simulink model "tuned"  (R2021a)
settings: Solver=VariableStepAuto  StartTime=0.0  StopTime=20  RelTol=1e-3
values from neighbouring files (symbols this model uses):
  A = processo.A    [esercizio1.m]
  B = processo.B    [esercizio1.m]
  C = processo.C    [esercizio1.m]
  D = processo.D    [esercizio1.m]
  I_PI_analogico_tuned = 0.325410877804267    (= 0.325410877804)    [esercizio1.m]
  I_PI_digitale_tuned = 0.28478840442912    (= 0.284788404429)    [esercizio1.m]
  I_PID_analogico_tuned = 0.279951410984123    (= 0.279951410984)    [esercizio1.m]
  I_PID_digitale_tuned = 0.172208500364823    (= 0.172208500365)    [esercizio1.m]
  KP_P = 0.5*Kcr    (= 2.15517241379)    [esercizio1.m]
  KP_P_analogico_tuned = 1.47219531686421    (= 1.47219531686)    [esercizio1.m]
  KP_P_digitale_tuned = 1.47219531686421    (= 1.47219531686)    [esercizio1.m]
  KP_PI = 0.45*Kcr    (= 1.93965517241)    [esercizio1.m]
  KP_PI_analogico_tuned = 1.47593963796892    (= 1.47593963797)    [esercizio1.m]
  KP_PI_digitale_tuned = 1.4003674925568    (= 1.40036749256)    [esercizio1.m]
  KP_PID = 0.6*Kcr    (= 2.58620689655)    [esercizio1.m]
  KP_PID_analogico_tuned = 1.9364815341473    (= 1.93648153415)    [esercizio1.m]
  KP_PID_digitale_tuned = 1.83497063890365    (= 1.8349706389)    [esercizio1.m]
  N = 100    [esercizio1.m]
  T = ta/40    [esercizio1.m]
  ta = 3*cost_temp_polo_dominante    [esercizio1.m]
  TD_PID = 0.12*Tcr    (= 0.24)    [esercizio1.m]
  TD_PID_analogico_tuned = 0.0554825984150835    (= 0.0554825984151)    [esercizio1.m]
  TD_PID_digitale_tuned = 0.0992484035615046    (= 0.0992484035615)    [esercizio1.m]
  TI_PI = 0.85*Tcr    (= 1.7)    [esercizio1.m]
  TI_PID = 0.5*Tcr    (= 1)    [esercizio1.m]
libraries: pid_lib x6
settings Model: Creator=Giorgio  LastModifiedBy=Giorgio

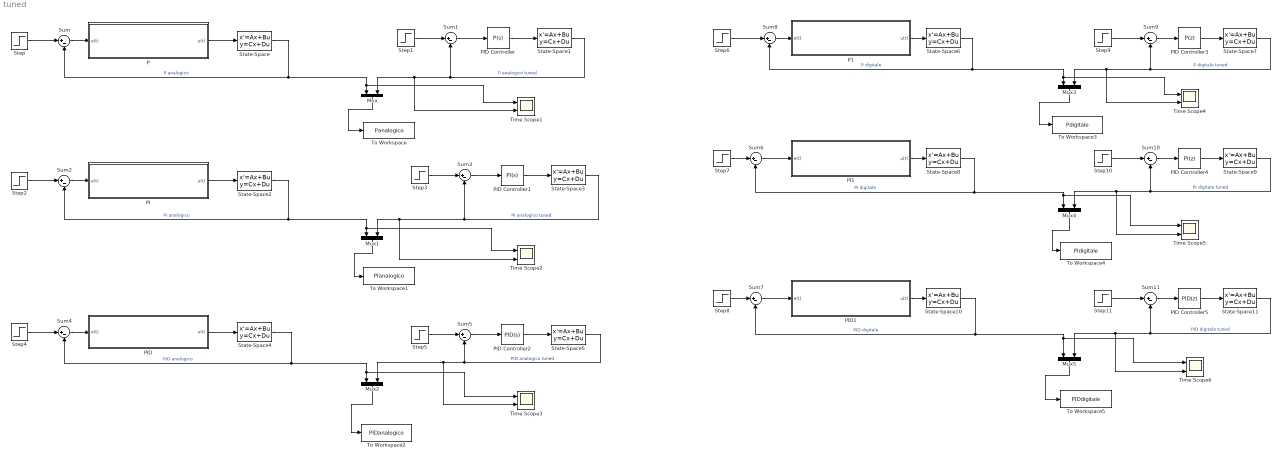
== system tuned ==
  Mux{,1..5} (6 alike) : Mux  Inputs=2
  P : Subsystem
  P1 : Subsystem
  PI : Subsystem
  PI1 : Subsystem
  PID : Subsystem
  PID Controller : pid_lib/PID Controller  Controller=P  Form=Ideal  TimeDomain=Continuous-time  UseExternalTs=off  SampleTime=-1  IntegratorMethod=Forward Euler  FilterMethod=Forward Euler  ControllerParametersSource=internal  P=KP_P_analogico_tuned  I=1  D=0  UseFilter=on  N=100  TunerSelectOption=Transfer Function Based (PID Tuner App)  InitialConditionSource=internal  InitialConditionForIntegrator=0  InitialConditionForFilter=0  DifferentiatorICPrevScaledInput=0  ExternalReset=none  TrackingMode=off  Kt=1  LimitOutput=off  SatLimitsSource=internal  UpperSaturationLimit=inf  LowerSaturationLimit=-inf  LinearizeAsGain=on  AntiWindupMode=none  Kb=1  POutMin=[]  POutMax=[]  IOutMin=[]  IOutMax=[]  DOutMin=[]  DOutMax=[]  NOutMin=[]  NOutMax=[]  SumOutMin=[]  SumOutMax=[]  SaturationOutMin=[]  SaturationOutMax=[]  PParamMin=[]  PParamMax=[]  IParamMin=[]  IParamMax=[]  DParamMin=[]  DParamMax=[]  NParamMin=[]  NParamMax=[]  KbParamMin=[]  KbParamMax=[]  KtParamMin=[]  KtParamMax=[]  KbOutMin=[]  KbOutMax=[]  KtOutMin=[]  KtOutMax=[]  IntegratorOutMin=[]  IntegratorOutMax=[]  FilterOutMin=[]  FilterOutMax=[]  SumI1OutMin=[]  SumI1OutMax=[]  SumI2OutMin=[]  SumI2OutMax=[]  SumI3OutMin=[]  SumI3OutMax=[]  SumI4OutMin=[]  SumI4OutMax=[]  SumDOutMin=[]  SumDOutMax=[]  DifferentiatorOutMin=[]  DifferentiatorOutMax=[]  FilterDiffOutCoefMin=[]  FilterDiffOutCoefMax=[]  ReciprocalOutMin=[]  ReciprocalOutMax=[]  SumDenOutMin=[]  SumDenOutMax=[]  SumNumOutMin=[]  SumNumOutMax=[]  DivideOutMin=[]  DivideOutMax=[]  UdiffTsProdOutMin=[]  UdiffTsProdOutMax=[]  NTsProdOutMin=[]  NTsProdOutMax=[]  UintegralTsProdOutMin=[]  UintegralTsProdOutMax=[]  UngainTsProdOutMin=[]  UngainTsProdOutMax=[]  IntegratorContinuousStateAttributes=''  IntegratorStateMustResolveToSignalObject=off  IntegratorRTWStateStorageClass=Auto  FilterContinuousStateAttributes=''  FilterStateMustResolveToSignalObject=off  FilterRTWStateStorageClass=Auto  ParallelPVariant=InternalParameters  IdealPVariant=Disabled  IVariant=Disabled  DVariant=Disabled  IntegratorVariant=Disabled  SatVariant=Disabled  AWVariant=Disabled  PCopyVariant=Disabled  TRVariant=Disabled  FdbkBlocksVariant=Forward  IdealPFdbkVariant=Disabled  SatFdbkVariant=Disabled  DerivativeFilterVariant=Disabled  NVariant=Disabled  NCopyVariant=Disabled_SignalSpec  FilterICVariant=Disabled  IntegratorICVariant=Disabled  ExternalResetVariant=Disabled  TRSumVariant=Passthrough  SumFdbkVariant=Disabled  SumVariant=Passthrough_P  TsampFilterVariant=InternalTs  TsampNgainVariant=Passthrough  TsampIntegralVariant=Disabled_SignalSpec  ExternalSaturationOutDataTypeStr=Inherit: Same as second input
  PID Controller1 : pid_lib/PID Controller  Controller=PI  Form=Ideal  TimeDomain=Continuous-time  UseExternalTs=off  SampleTime=-1  IntegratorMethod=Forward Euler  FilterMethod=Forward Euler  ControllerParametersSource=internal  P=KP_PI_analogico_tuned  I=I_PI_analogico_tuned  D=0  UseFilter=on  N=100  TunerSelectOption=Transfer Function Based (PID Tuner App)  InitialConditionSource=internal  InitialConditionForIntegrator=0  InitialConditionForFilter=0  DifferentiatorICPrevScaledInput=0  ExternalReset=none  TrackingMode=off  Kt=1  LimitOutput=off  SatLimitsSource=internal  UpperSaturationLimit=inf  LowerSaturationLimit=-inf  LinearizeAsGain=on  AntiWindupMode=none  Kb=1  POutMin=[]  POutMax=[]  IOutMin=[]  IOutMax=[]  DOutMin=[]  DOutMax=[]  NOutMin=[]  NOutMax=[]  SumOutMin=[]  SumOutMax=[]  SaturationOutMin=[]  SaturationOutMax=[]  PParamMin=[]  PParamMax=[]  IParamMin=[]  IParamMax=[]  DParamMin=[]  DParamMax=[]  NParamMin=[]  NParamMax=[]  KbParamMin=[]  KbParamMax=[]  KtParamMin=[]  KtParamMax=[]  KbOutMin=[]  KbOutMax=[]  KtOutMin=[]  KtOutMax=[]  IntegratorOutMin=[]  IntegratorOutMax=[]  FilterOutMin=[]  FilterOutMax=[]  SumI1OutMin=[]  SumI1OutMax=[]  SumI2OutMin=[]  SumI2OutMax=[]  SumI3OutMin=[]  SumI3OutMax=[]  SumI4OutMin=[]  SumI4OutMax=[]  SumDOutMin=[]  SumDOutMax=[]  DifferentiatorOutMin=[]  DifferentiatorOutMax=[]  FilterDiffOutCoefMin=[]  FilterDiffOutCoefMax=[]  ReciprocalOutMin=[]  ReciprocalOutMax=[]  SumDenOutMin=[]  SumDenOutMax=[]  SumNumOutMin=[]  SumNumOutMax=[]  DivideOutMin=[]  DivideOutMax=[]  UdiffTsProdOutMin=[]  UdiffTsProdOutMax=[]  NTsProdOutMin=[]  NTsProdOutMax=[]  UintegralTsProdOutMin=[]  UintegralTsProdOutMax=[]  UngainTsProdOutMin=[]  UngainTsProdOutMax=[]  IntegratorContinuousStateAttributes=''  IntegratorStateMustResolveToSignalObject=off  IntegratorRTWStateStorageClass=Auto  FilterContinuousStateAttributes=''  FilterStateMustResolveToSignalObject=off  FilterRTWStateStorageClass=Auto  ParallelPVariant=Passthrough  IdealPVariant=InternalParameters  IVariant=InternalParameters  DVariant=Disabled  IntegratorVariant=Continuous  SatVariant=Disabled  AWVariant=Passthrough  PCopyVariant=Disabled  TRVariant=Disabled  FdbkBlocksVariant=Forward  IdealPFdbkVariant=Disabled  SatFdbkVariant=Disabled  DerivativeFilterVariant=Disabled  NVariant=Disabled  NCopyVariant=Disabled_SignalSpec  FilterICVariant=Disabled  IntegratorICVariant=InternalICs  ExternalResetVariant=Disabled  TRSumVariant=Passthrough  SumFdbkVariant=Disabled  SumVariant=Sum_PI  TsampFilterVariant=InternalTs  TsampNgainVariant=Passthrough  TsampIntegralVariant=Passthrough  ExternalSaturationOutDataTypeStr=Inherit: Same as second input
  PID Controller2 : pid_lib/PID Controller  Controller=PID  Form=Ideal  TimeDomain=Continuous-time  UseExternalTs=off  SampleTime=-1  IntegratorMethod=Forward Euler  FilterMethod=Forward Euler  ControllerParametersSource=internal  P=KP_PID_analogico_tuned  I=I_PID_analogico_tuned  D=TD_PID_analogico_tuned  UseFilter=on  N=N  TunerSelectOption=Transfer Function Based (PID Tuner App)  InitialConditionSource=internal  InitialConditionForIntegrator=0  InitialConditionForFilter=0  DifferentiatorICPrevScaledInput=0  ExternalReset=none  TrackingMode=off  Kt=1  LimitOutput=off  SatLimitsSource=internal  UpperSaturationLimit=inf  LowerSaturationLimit=-inf  LinearizeAsGain=on  AntiWindupMode=none  Kb=1  POutMin=[]  POutMax=[]  IOutMin=[]  IOutMax=[]  DOutMin=[]  DOutMax=[]  NOutMin=[]  NOutMax=[]  SumOutMin=[]  SumOutMax=[]  SaturationOutMin=[]  SaturationOutMax=[]  PParamMin=[]  PParamMax=[]  IParamMin=[]  IParamMax=[]  DParamMin=[]  DParamMax=[]  NParamMin=[]  NParamMax=[]  KbParamMin=[]  KbParamMax=[]  KtParamMin=[]  KtParamMax=[]  KbOutMin=[]  KbOutMax=[]  KtOutMin=[]  KtOutMax=[]  IntegratorOutMin=[]  IntegratorOutMax=[]  FilterOutMin=[]  FilterOutMax=[]  SumI1OutMin=[]  SumI1OutMax=[]  SumI2OutMin=[]  SumI2OutMax=[]  SumI3OutMin=[]  SumI3OutMax=[]  SumI4OutMin=[]  SumI4OutMax=[]  SumDOutMin=[]  SumDOutMax=[]  DifferentiatorOutMin=[]  DifferentiatorOutMax=[]  FilterDiffOutCoefMin=[]  FilterDiffOutCoefMax=[]  ReciprocalOutMin=[]  ReciprocalOutMax=[]  SumDenOutMin=[]  SumDenOutMax=[]  SumNumOutMin=[]  SumNumOutMax=[]  DivideOutMin=[]  DivideOutMax=[]  UdiffTsProdOutMin=[]  UdiffTsProdOutMax=[]  NTsProdOutMin=[]  NTsProdOutMax=[]  UintegralTsProdOutMin=[]  UintegralTsProdOutMax=[]  UngainTsProdOutMin=[]  UngainTsProdOutMax=[]  IntegratorContinuousStateAttributes=''  IntegratorStateMustResolveToSignalObject=off  IntegratorRTWStateStorageClass=Auto  FilterContinuousStateAttributes=''  FilterStateMustResolveToSignalObject=off  FilterRTWStateStorageClass=Auto  ParallelPVariant=Passthrough  IdealPVariant=InternalParameters  IVariant=InternalParameters  DVariant=InternalParameters  IntegratorVariant=Continuous  SatVariant=Disabled  AWVariant=Passthrough  PCopyVariant=Disabled  TRVariant=Disabled  FdbkBlocksVariant=Forward  IdealPFdbkVariant=Disabled  SatFdbkVariant=Disabled  DerivativeFilterVariant=ContFilter  NVariant=InternalParameters  NCopyVariant=Disabled  FilterICVariant=InternalICsFilter  IntegratorICVariant=InternalICs  ExternalResetVariant=Disabled  TRSumVariant=Passthrough  SumFdbkVariant=Disabled  SumVariant=Sum_PID  TsampFilterVariant=InternalTs  TsampNgainVariant=Passthrough  TsampIntegralVariant=Passthrough  ExternalSaturationOutDataTypeStr=Inherit: Same as second input
  PID Controller3 : pid_lib/PID Controller  Controller=P  Form=Parallel  TimeDomain=Discrete-time  UseExternalTs=off  SampleTime=-1  IntegratorMethod=Forward Euler  FilterMethod=Forward Euler  ControllerParametersSource=internal  P=KP_P_digitale_tuned  I=1  D=0  UseFilter=on  N=100  TunerSelectOption=Transfer Function Based (PID Tuner App)  InitialConditionSource=internal  InitialConditionForIntegrator=0  InitialConditionForFilter=0  DifferentiatorICPrevScaledInput=0  ExternalReset=none  TrackingMode=off  Kt=1  LimitOutput=off  SatLimitsSource=internal  UpperSaturationLimit=inf  LowerSaturationLimit=-inf  LinearizeAsGain=on  AntiWindupMode=none  Kb=1  POutMin=[]  POutMax=[]  IOutMin=[]  IOutMax=[]  DOutMin=[]  DOutMax=[]  NOutMin=[]  NOutMax=[]  SumOutMin=[]  SumOutMax=[]  SaturationOutMin=[]  SaturationOutMax=[]  PParamMin=[]  PParamMax=[]  IParamMin=[]  IParamMax=[]  DParamMin=[]  DParamMax=[]  NParamMin=[]  NParamMax=[]  KbParamMin=[]  KbParamMax=[]  KtParamMin=[]  KtParamMax=[]  KbOutMin=[]  KbOutMax=[]  KtOutMin=[]  KtOutMax=[]  IntegratorOutMin=[]  IntegratorOutMax=[]  FilterOutMin=[]  FilterOutMax=[]  SumI1OutMin=[]  SumI1OutMax=[]  SumI2OutMin=[]  SumI2OutMax=[]  SumI3OutMin=[]  SumI3OutMax=[]  SumI4OutMin=[]  SumI4OutMax=[]  SumDOutMin=[]  SumDOutMax=[]  DifferentiatorOutMin=[]  DifferentiatorOutMax=[]  FilterDiffOutCoefMin=[]  FilterDiffOutCoefMax=[]  ReciprocalOutMin=[]  ReciprocalOutMax=[]  SumDenOutMin=[]  SumDenOutMax=[]  SumNumOutMin=[]  SumNumOutMax=[]  DivideOutMin=[]  DivideOutMax=[]  UdiffTsProdOutMin=[]  UdiffTsProdOutMax=[]  NTsProdOutMin=[]  NTsProdOutMax=[]  UintegralTsProdOutMin=[]  UintegralTsProdOutMax=[]  UngainTsProdOutMin=[]  UngainTsProdOutMax=[]  IntegratorContinuousStateAttributes=''  IntegratorStateMustResolveToSignalObject=off  IntegratorRTWStateStorageClass=Auto  FilterContinuousStateAttributes=''  FilterStateMustResolveToSignalObject=off  FilterRTWStateStorageClass=Auto  ParallelPVariant=InternalParameters  IdealPVariant=Disabled  IVariant=Disabled  DVariant=Disabled  IntegratorVariant=Disabled  SatVariant=Disabled  AWVariant=Disabled  PCopyVariant=Disabled  TRVariant=Disabled  FdbkBlocksVariant=Forward  IdealPFdbkVariant=Disabled  SatFdbkVariant=Disabled  DerivativeFilterVariant=Disabled  NVariant=Disabled  NCopyVariant=Disabled_SignalSpec  FilterICVariant=Disabled  IntegratorICVariant=Disabled  ExternalResetVariant=Disabled  TRSumVariant=Passthrough  SumFdbkVariant=Disabled  SumVariant=Passthrough_P  TsampFilterVariant=InternalTs  TsampNgainVariant=Passthrough  TsampIntegralVariant=Disabled_SignalSpec  ExternalSaturationOutDataTypeStr=Inherit: Same as second input
  PID Controller4 : pid_lib/PID Controller  Controller=PI  Form=Ideal  TimeDomain=Discrete-time  UseExternalTs=off  SampleTime=-1  IntegratorMethod=Trapezoidal  FilterMethod=Forward Euler  ControllerParametersSource=internal  P=KP_PI_digitale_tuned  I=I_PI_digitale_tuned  D=0  UseFilter=on  N=100  TunerSelectOption=Transfer Function Based (PID Tuner App)  InitialConditionSource=internal  InitialConditionForIntegrator=0  InitialConditionForFilter=0  DifferentiatorICPrevScaledInput=0  ExternalReset=none  TrackingMode=off  Kt=1  LimitOutput=off  SatLimitsSource=internal  UpperSaturationLimit=inf  LowerSaturationLimit=-inf  LinearizeAsGain=on  AntiWindupMode=none  Kb=1  POutMin=[]  POutMax=[]  IOutMin=[]  IOutMax=[]  DOutMin=[]  DOutMax=[]  NOutMin=[]  NOutMax=[]  SumOutMin=[]  SumOutMax=[]  SaturationOutMin=[]  SaturationOutMax=[]  PParamMin=[]  PParamMax=[]  IParamMin=[]  IParamMax=[]  DParamMin=[]  DParamMax=[]  NParamMin=[]  NParamMax=[]  KbParamMin=[]  KbParamMax=[]  KtParamMin=[]  KtParamMax=[]  KbOutMin=[]  KbOutMax=[]  KtOutMin=[]  KtOutMax=[]  IntegratorOutMin=[]  IntegratorOutMax=[]  FilterOutMin=[]  FilterOutMax=[]  SumI1OutMin=[]  SumI1OutMax=[]  SumI2OutMin=[]  SumI2OutMax=[]  SumI3OutMin=[]  SumI3OutMax=[]  SumI4OutMin=[]  SumI4OutMax=[]  SumDOutMin=[]  SumDOutMax=[]  DifferentiatorOutMin=[]  DifferentiatorOutMax=[]  FilterDiffOutCoefMin=[]  FilterDiffOutCoefMax=[]  ReciprocalOutMin=[]  ReciprocalOutMax=[]  SumDenOutMin=[]  SumDenOutMax=[]  SumNumOutMin=[]  SumNumOutMax=[]  DivideOutMin=[]  DivideOutMax=[]  UdiffTsProdOutMin=[]  UdiffTsProdOutMax=[]  NTsProdOutMin=[]  NTsProdOutMax=[]  UintegralTsProdOutMin=[]  UintegralTsProdOutMax=[]  UngainTsProdOutMin=[]  UngainTsProdOutMax=[]  IntegratorContinuousStateAttributes=''  IntegratorStateMustResolveToSignalObject=off  IntegratorRTWStateStorageClass=Auto  FilterContinuousStateAttributes=''  FilterStateMustResolveToSignalObject=off  FilterRTWStateStorageClass=Auto  ParallelPVariant=Passthrough  IdealPVariant=InternalParameters  IVariant=InternalParameters  DVariant=Disabled  IntegratorVariant=Discrete  SatVariant=Disabled  AWVariant=Passthrough  PCopyVariant=Disabled  TRVariant=Disabled  FdbkBlocksVariant=Forward  IdealPFdbkVariant=Disabled  SatFdbkVariant=Disabled  DerivativeFilterVariant=Disabled  NVariant=Disabled  NCopyVariant=Disabled_SignalSpec  FilterICVariant=Disabled  IntegratorICVariant=InternalICs  ExternalResetVariant=Disabled  TRSumVariant=Passthrough  SumFdbkVariant=Disabled  SumVariant=Sum_PI  TsampFilterVariant=InternalTs  TsampNgainVariant=Passthrough  TsampIntegralVariant=Passthrough  ExternalSaturationOutDataTypeStr=Inherit: Same as second input
  PID Controller5 : pid_lib/PID Controller  Controller=PID  Form=Ideal  TimeDomain=Discrete-time  UseExternalTs=off  SampleTime=-1  IntegratorMethod=Trapezoidal  FilterMethod=Trapezoidal  ControllerParametersSource=internal  P=KP_PID_digitale_tuned  I=I_PID_digitale_tuned  D=TD_PID_digitale_tuned  UseFilter=on  N=N  TunerSelectOption=Transfer Function Based (PID Tuner App)  InitialConditionSource=internal  InitialConditionForIntegrator=0  InitialConditionForFilter=0  DifferentiatorICPrevScaledInput=0  ExternalReset=none  TrackingMode=off  Kt=1  LimitOutput=off  SatLimitsSource=internal  UpperSaturationLimit=inf  LowerSaturationLimit=-inf  LinearizeAsGain=on  AntiWindupMode=none  Kb=1  POutMin=[]  POutMax=[]  IOutMin=[]  IOutMax=[]  DOutMin=[]  DOutMax=[]  NOutMin=[]  NOutMax=[]  SumOutMin=[]  SumOutMax=[]  SaturationOutMin=[]  SaturationOutMax=[]  PParamMin=[]  PParamMax=[]  IParamMin=[]  IParamMax=[]  DParamMin=[]  DParamMax=[]  NParamMin=[]  NParamMax=[]  KbParamMin=[]  KbParamMax=[]  KtParamMin=[]  KtParamMax=[]  KbOutMin=[]  KbOutMax=[]  KtOutMin=[]  KtOutMax=[]  IntegratorOutMin=[]  IntegratorOutMax=[]  FilterOutMin=[]  FilterOutMax=[]  SumI1OutMin=[]  SumI1OutMax=[]  SumI2OutMin=[]  SumI2OutMax=[]  SumI3OutMin=[]  SumI3OutMax=[]  SumI4OutMin=[]  SumI4OutMax=[]  SumDOutMin=[]  SumDOutMax=[]  DifferentiatorOutMin=[]  DifferentiatorOutMax=[]  FilterDiffOutCoefMin=[]  FilterDiffOutCoefMax=[]  ReciprocalOutMin=[]  ReciprocalOutMax=[]  SumDenOutMin=[]  SumDenOutMax=[]  SumNumOutMin=[]  SumNumOutMax=[]  DivideOutMin=[]  DivideOutMax=[]  UdiffTsProdOutMin=[]  UdiffTsProdOutMax=[]  NTsProdOutMin=[]  NTsProdOutMax=[]  UintegralTsProdOutMin=[]  UintegralTsProdOutMax=[]  UngainTsProdOutMin=[]  UngainTsProdOutMax=[]  IntegratorContinuousStateAttributes=''  IntegratorStateMustResolveToSignalObject=off  IntegratorRTWStateStorageClass=Auto  FilterContinuousStateAttributes=''  FilterStateMustResolveToSignalObject=off  FilterRTWStateStorageClass=Auto  ParallelPVariant=Passthrough  IdealPVariant=InternalParameters  IVariant=InternalParameters  DVariant=InternalParameters  IntegratorVariant=Discrete  SatVariant=Disabled  AWVariant=Passthrough  PCopyVariant=Disabled  TRVariant=Disabled  FdbkBlocksVariant=Forward  IdealPFdbkVariant=Disabled  SatFdbkVariant=Disabled  DerivativeFilterVariant=TrapezoidalFilter  NVariant=InternalParameters  NCopyVariant=InternalParameters  FilterICVariant=InternalICsFilter  IntegratorICVariant=InternalICs  ExternalResetVariant=Disabled  TRSumVariant=Passthrough  SumFdbkVariant=Disabled  SumVariant=Sum_PID  TsampFilterVariant=InternalTs  TsampNgainVariant=Passthrough  TsampIntegralVariant=Passthrough  ExternalSaturationOutDataTypeStr=Inherit: Same as second input
  PID1 : Subsystem
  State-Space{,1..11} (12 alike) : StateSpace  A=A  B=B  C=C  D=D  InitialCondition=0
  Step{,1..11} (12 alike) : Step  Time=0  SampleTime=0
  Sum{,1..11} (12 alike) : Sum  Inputs=|+-
  Time Scope{1..6} (6 alike) : Scope  NumInputPorts=2
  To Workspace : ToWorkspace  VariableName=Panalogico  SaveFormat=Timeseries  SampleTime=-1
  To Workspace1 : ToWorkspace  VariableName=PIanalogico  SaveFormat=Timeseries  SampleTime=-1
  To Workspace2 : ToWorkspace  VariableName=PIDanalogico  SaveFormat=Timeseries  SampleTime=-1
  To Workspace3 : ToWorkspace  VariableName=Pdigitale  SaveFormat=Timeseries  SampleTime=-1
  To Workspace4 : ToWorkspace  VariableName=PIdigitale  SaveFormat=Timeseries  SampleTime=-1
  To Workspace5 : ToWorkspace  VariableName=PIDdigitale  SaveFormat=Timeseries  SampleTime=-1
  wires:
  Sum2/1 -> PI/1(e(t))
  P/1(u(t)) -> State-Space/1
  PID/1(u(t)) -> State-Space4/1
  PI/1(u(t)) -> State-Space2/1
  Sum/1 -> P/1(e(t))
  Sum4/1 -> PID/1(e(t))
  State-Space4/1 -> Time Scope3/1, Mux2/1, Sum4/2  "PID analogico"
  State-Space5/1 -> Sum5/2, Time Scope3/2, Mux2/2  "PID analogico tuned"
  Mux1/1 -> To Workspace1/1
  State-Space/1 -> Sum/2, Time Scope1/1, Mux/1  "P analogico"
  Step5/1 -> Sum5/1
  PID Controller2/1 -> State-Space5/1
  State-Space1/1 -> Sum1/2, Time Scope1/2, Mux/2  "P analogico tuned"
  PID Controller1/1 -> State-Space3/1
  Step/1 -> Sum/1
  Step3/1 -> Sum3/1
  Mux/1 -> To Workspace/1
  Sum1/1 -> PID Controller/1
  Step4/1 -> Sum4/1
  Step1/1 -> Sum1/1
  Step2/1 -> Sum2/1
  State-Space2/1 -> Sum2/2, Time Scope2/1, Mux1/1  "PI analogico"
  State-Space3/1 -> Sum3/2, Time Scope2/2, Mux1/2  "PI analogico tuned"
  Sum5/1 -> PID Controller2/1
  Mux2/1 -> To Workspace2/1
  PID Controller/1 -> State-Space1/1
  Sum3/1 -> PID Controller1/1
  State-Space9/1 -> Sum10/2, Time Scope5/2, Mux4/2  "PI digitale tuned"
  State-Space6/1 -> Sum8/2, Time Scope4/1, Mux3/1  "P digitale"
  State-Space8/1 -> Time Scope5/1, Mux4/1, Sum6/2  "PI digitale"
  PID Controller3/1 -> State-Space7/1
  Step7/1 -> Sum6/1
  Mux3/1 -> To Workspace3/1
  Sum9/1 -> PID Controller3/1
  Step6/1 -> Sum8/1
  State-Space11/1 -> Sum11/2, Time Scope6/2, Mux5/2  "PID digitale tuned"
  Step10/1 -> Sum10/1
  State-Space10/1 -> Sum7/2, Time Scope6/1, Mux5/1  "PID digitale"
  PID Controller4/1 -> State-Space9/1
  Mux4/1 -> To Workspace4/1
  Step11/1 -> Sum11/1
  PI1/1(u(t)) -> State-Space8/1
  Sum8/1 -> P1/1(e(t))
  PID Controller5/1 -> State-Space11/1
  Step8/1 -> Sum7/1
  Sum7/1 -> PID1/1(e(t))
  P1/1(u(t)) -> State-Space6/1
  Mux5/1 -> To Workspace5/1
  Sum10/1 -> PID Controller4/1
  Sum6/1 -> PI1/1(e(t))
  PID1/1(u(t)) -> State-Space10/1
  State-Space7/1 -> Sum9/2, Time Scope4/2, Mux3/2  "P digitale tuned"
  Sum11/1 -> PID Controller5/1
  Step9/1 -> Sum9/1

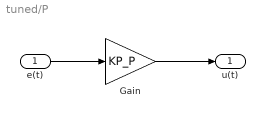
== system tuned/P ==
  e(t) : Inport
  Gain : Gain  Gain=KP_P
  u(t) : Outport
  wires:
  Gain/1 -> u(t)/1
  e(t)/1 -> Gain/1

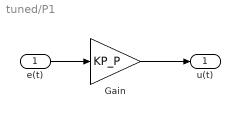
== system tuned/P1 ==
  e(t) : Inport
  Gain : Gain  Gain=KP_P
  u(t) : Outport
  wires:
  e(t)/1 -> Gain/1
  Gain/1 -> u(t)/1

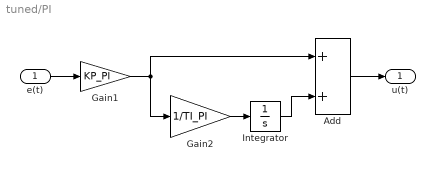
== system tuned/PI ==
  e(t) : Inport
  Add : Sum
  Gain1 : Gain  Gain=KP_PI
  Gain2 : Gain  Gain=1/TI_PI
  Integrator : Integrator
  u(t) : Outport
  wires:
  Add/1 -> u(t)/1
  Gain1/1 -> Add/1, Gain2/1
  Integrator/1 -> Add/2
  Gain2/1 -> Integrator/1
  e(t)/1 -> Gain1/1

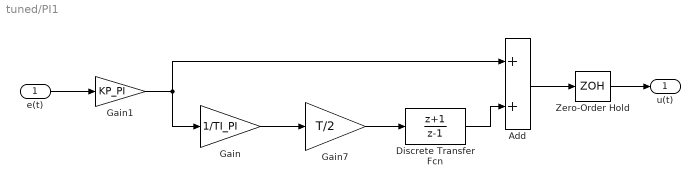
== system tuned/PI1 ==
  e(t) : Inport
  Add : Sum
  Discrete Transfer Fcn : DiscreteTransferFcn  Numerator=[1 1]  Denominator=[1 -1]
  Gain : Gain  Gain=1/TI_PI
  Gain1 : Gain  Gain=KP_PI
  Gain7 : Gain  Gain=T/2
  Zero-Order Hold : ZeroOrderHold  SampleTime=ta/40
  u(t) : Outport
  wires:
  Gain1/1 -> Add/1, Gain/1
  Gain7/1 -> Discrete Transfer Fcn/1
  Gain/1 -> Gain7/1
  Add/1 -> Zero-Order Hold/1
  Zero-Order Hold/1 -> u(t)/1
  Discrete Transfer Fcn/1 -> Add/2
  e(t)/1 -> Gain1/1

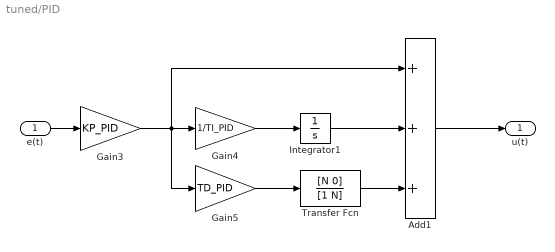
== system tuned/PID ==
  e(t) : Inport
  Add1 : Sum  Inputs=+++
  Gain3 : Gain  Gain=KP_PID
  Gain4 : Gain  Gain=1/TI_PID
  Gain5 : Gain  Gain=TD_PID
  Integrator1 : Integrator
  Transfer Fcn : TransferFcn  Numerator=[N 0]  Denominator=[1 N]
  u(t) : Outport
  wires:
  Gain5/1 -> Transfer Fcn/1
  Transfer Fcn/1 -> Add1/3
  Gain4/1 -> Integrator1/1
  Add1/1 -> u(t)/1
  Gain3/1 -> Gain5/1, Add1/1, Gain4/1
  Integrator1/1 -> Add1/2
  e(t)/1 -> Gain3/1

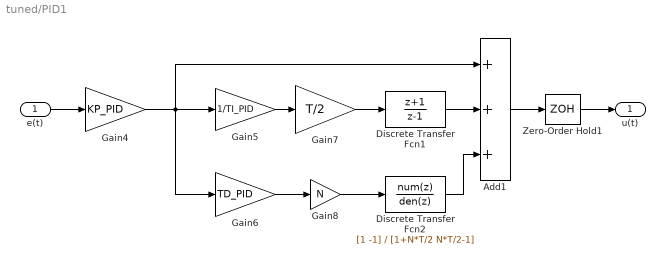
== system tuned/PID1 ==
  e(t) : Inport
  Add1 : Sum  Inputs=+++
  Discrete Transfer Fcn1 : DiscreteTransferFcn  Numerator=[1 1]  Denominator=[1 -1]
  Discrete Transfer Fcn2 : DiscreteTransferFcn  Numerator=[1 -1]  Denominator=[1+N*T/2 N*T/2-1]
  Gain4 : Gain  Gain=KP_PID
  Gain5 : Gain  Gain=1/TI_PID
  Gain6 : Gain  Gain=TD_PID
  Gain7 : Gain  Gain=T/2
  Gain8 : Gain  Gain=N
  Zero-Order Hold1 : ZeroOrderHold  SampleTime=T
  u(t) : Outport
  wires:
  Gain7/1 -> Discrete Transfer Fcn1/1
  Discrete Transfer Fcn2/1 -> Add1/3
  Gain6/1 -> Gain8/1
  Add1/1 -> Zero-Order Hold1/1
  Gain5/1 -> Gain7/1
  Gain8/1 -> Discrete Transfer Fcn2/1
  Gain4/1 -> Gain6/1, Gain5/1, Add1/1
  Discrete Transfer Fcn1/1 -> Add1/2
  e(t)/1 -> Gain4/1
  Zero-Order Hold1/1 -> u(t)/1
